simulink model "StateMachineModel"  (R2020a)
settings: Solver=VariableStepAuto  StartTime=0.0  StopTime=10.0  RelTol=1e-3
settings Model: Creator=pedro  LastModifiedBy=pedro

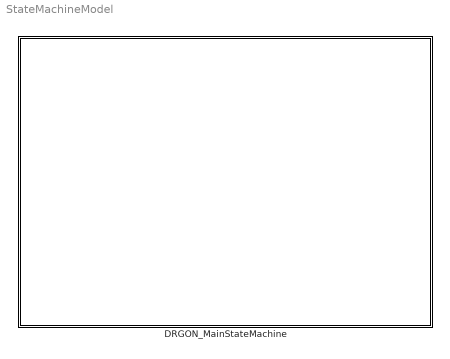
== system StateMachineModel ==
  DRGON_MainStateMachine : Stateflow chart  TreatAsAtomicUnit=on

== stateflow chart StateMachineModel/DRGON_MainStateMachine ==
  state Standby
  state Respiration
    state ForcedVolumeBased
      state GenerateTrajectory
      state Pause
      state Inhale
      state Exhale
      (default) -> Respiration.ForcedVolumeBased.GenerateTrajectory : {ReadParams}
      Respiration.ForcedVolumeBased.GenerateTrajectory -> Respiration.ForcedVolumeBased.Inhale : [TrajectoryDone]
      Respiration.ForcedVolumeBased.Inhale -> Respiration.ForcedVolumeBased.Pause : [VolReached]
      Respiration.ForcedVolumeBased.Exhale -> Respiration.ForcedVolumeBased.Inhale : [OriginReached]
      Respiration.ForcedVolumeBased.Pause -> Respiration.ForcedVolumeBased.Exhale : [PauseTimeElapsed]
    state AssistedVolumeBased
      state GenerateTrajectory
      state Inhale
      state WaitForInhalation
      state Pause
      state Exhale
      (default) -> Respiration.AssistedVolumeBased.GenerateTrajectory : {ReadParams}
      Respiration.AssistedVolumeBased.GenerateTrajectory -> WaitForInhalation : [TrajectoryDone]
      WaitForInhalation -> Respiration.AssistedVolumeBased.Inhale : [PatientInhaled || TimeoutElapsed]
      Respiration.AssistedVolumeBased.Exhale -> WaitForInhalation : [OriginReached]
      Respiration.AssistedVolumeBased.Inhale -> Respiration.AssistedVolumeBased.Pause : [VolReached]
      Respiration.AssistedVolumeBased.Pause -> Respiration.AssistedVolumeBased.Exhale : [PauseTimeElapsed]
    (default) -> (junction 9) : {ReadMode}
    (junction 9) -> (junction 10) [order 2]
    (junction 9) -> ForcedVolumeBased [order 1] : [Mode == ForcedVolumeBased]
    (junction 10) -> AssistedVolumeBased
  state Setup
    state Standby
    state Calibration
      state CW
        TurnMotor CW
      state STOP_WAIT
        StopMotor
      state CCW
        TurnMotor CCW
      state STOP_DONE
        StopMotor
        Set Encoders to 0
        CalibEnded = 1
      (default) -> Setup.Calibration.CW
      Setup.Calibration.CW -> STOP_WAIT : [UnwindTiElapsed]
      STOP_WAIT -> Setup.Calibration.CCW : [CalibBtnPressed]
      Setup.Calibration.CCW -> STOP_DONE : [ArmEncMoves]
    state ManualSpin
      state Stop
      state CW
      state CCW
      (default) -> Stop
      Stop -> Setup.ManualSpin.CW : [EditBtnPressed]
      Setup.ManualSpin.CCW -> Stop : [EditBtnPressed]
      Setup.ManualSpin.CW -> Setup.ManualSpin.CCW : [EditBtnPressed]
    (default) -> Setup.Standby
    Setup.Standby -> Calibration [order 1] : [CalibBtnPressed]
    Setup.Standby -> ManualSpin [order 2] : [EditBtnPressed]
  (default) -> Standby
  Respiration -> Standby : [StartBtnPressed && RoutineOn]
  Setup -> Standby : [StartBtnPressed || CalibEnded]
      | {CalibEnded = 0}
  Standby -> Respiration [order 2] : [StartBtnpressed && RoutineNotOn]
  Standby -> Setup [order 1] : [CalibBtnPressed && RoutineNotOn]
